simulink model "massamola_R14"  (Simulink 6.3)
settings: Solver=ode45  StartTime=0.0  StopTime=50.0  RelTol=1e-3
libraries: simulink x1
settings Model: LastModifiedBy=lucas

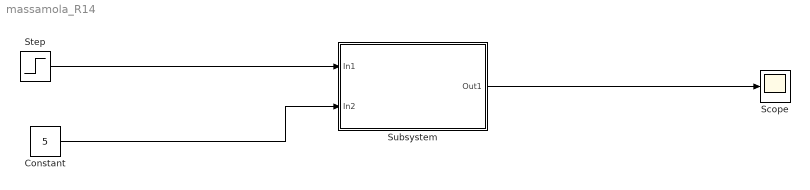
== system massamola_R14 ==
  Constant : Constant  Value=5
  Scope : Scope
  Step : Step  SampleTime=0
  Subsystem : Subsystem
  wires:
  Constant/1 -> Subsystem/2(In2)
  Subsystem/1(Out1) -> Scope/1
  Step/1 -> Subsystem/1(In1)

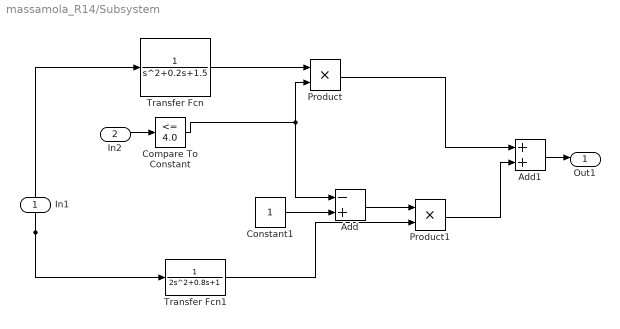
== system massamola_R14/Subsystem ==
  In1 : Inport  Orientation=down
  In2 : Inport  Port=2
  Add : Sum  Inputs=-+  OutScaling=2^-10
  Add1 : Sum  OutScaling=2^-10
  Compare To Constant : simulink/Logic and Bit Operations/Compare To Constant  relop=<=  const=4.0  LogicOutDataTypeMode=uint8  ZeroCross=off
  Constant1 : Constant
  Product : Product  RndMeth=Zero
  Product1 : Product  RndMeth=Zero
  Transfer Fcn : TransferFcn  Numerator=1  Denominator=[1 0.2 1.5]
  Transfer Fcn1 : TransferFcn  Numerator=1  Denominator=[2 0.8 1]
  Out1 : Outport
  wires:
  In1/1 -> Transfer Fcn1/1, Transfer Fcn/1
  Compare To Constant/1 -> Product/2, Add/1
  Transfer Fcn/1 -> Product/1
  Constant1/1 -> Add/2
  Add/1 -> Product1/1
  Transfer Fcn1/1 -> Product1/2
  Product/1 -> Add1/1
  Product1/1 -> Add1/2
  In2/1 -> Compare To Constant/1
  Add1/1 -> Out1/1
